simulink library "nmc"  (R2017b)
settings: Solver=ode45  StartTime=0.0  StopTime=10.0  RelTol=1e-3
undefined symbols (not defined in the file or in its folder): GroundFunction, theta
libraries: simulink x1
settings Model: Creator=efx  LastModifiedBy=FluitR
settings DataIOCC: LimitDataPoints=on  SaveFormat=Array
settings OptimizationCC: BlockReduction=off  BooleanDataType=off  LifeSpan=inf
settings DebuggingCC: SaveWithParameterizedLinksMsg=none  UnderspecifiedInitializationDetection=Classic  MergeDetectMultiDrivingBlocksExec=none  SignalResolutionControl=TryResolveAllWithWarning  AllowSymbolicDim=off  StrictBusMsg=Warning  SFUnexpectedBacktrackingDiag=warning  SFNoUnconditionalDefaultTransitionDiag=warning  SFExecutionAtInitializationDiag=none
settings HardwareCC: ProdBitPerPointer=32  ProdBitPerSizeT=32  ProdBitPerPtrDiffT=32  ProdLargestAtomicFloat=None  ProdIntDivRoundTo=Undefined  ProdEndianess=Unspecified  ProdWordSize=32  ProdHWDeviceType=32-bit Generic  TargetUnknown=on
settings ModelReferenceCC: PropagateSignalLabelsOutOfModel=off
settings CodeAppCC: StateflowObjectComments=on
settings GRTTargetCC: TargetLangStandard=C89/C90 (ANSI)  GeneratePreprocessorConditionals=Disable all
settings ConfigComp: CovMetricSettings=dw  CovHtmlReporting=on  CovSaveCumulativeToWorkspaceVar=on  CovSaveSingleToWorkspaceVar=on  CovExternalEMLEnable=off  CovSFcnEnable=off

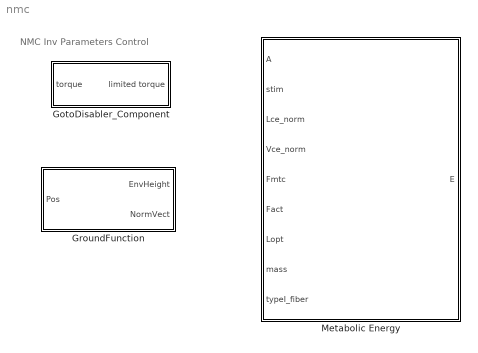
== system nmc ==
  note: NMC Inv Parameters Control
  GotoDisabler_Component : Subsystem  mask{GotoTag=DisableNMC_Component}
      mask prompts: GotoTag "Simulink:blkprm_prompts:FromGotoTag"
      mask TypeOptions GotoTag: From/GotoTag
      mask DialogControl GotoTag Prompt: Goto tag:
  GroundFunction : Subsystem
  Metabolic Energy : MATLAB Function  TreatAsAtomicUnit=on

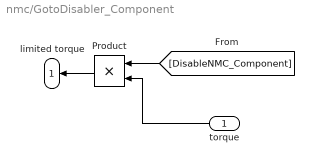
== system nmc/GotoDisabler_Component ==
  torque : Inport
  Product : Product
  limited torque : Outport
  wires:
  [DisableNMC_Component] -> Product/1
  Product/1 -> limited torque/1
  torque/1 -> Product/2

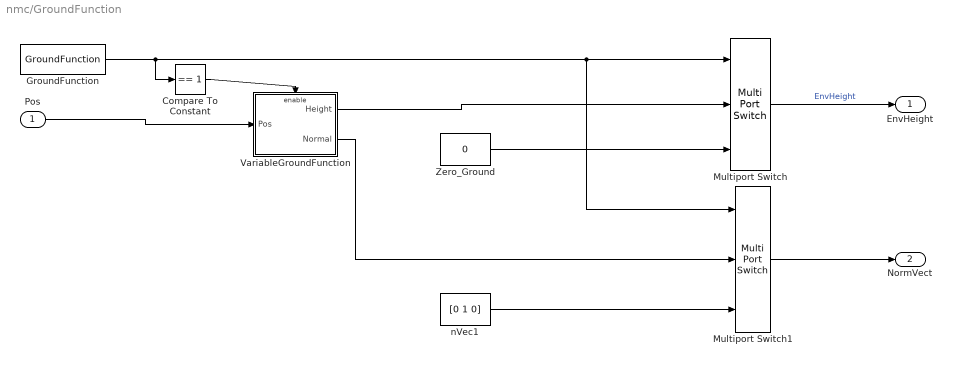
== system nmc/GroundFunction ==
  Pos : Inport
  Compare To Constant : simulink/Logic and Bit Operations/Compare To Constant  relop===  const=1  OutDataTypeStr=boolean  ZeroCross=off
  GroundFunction : Constant  Value=GroundFunction
  Multiport Switch : MultiPortSwitch  Inputs=2
  Multiport Switch1 : MultiPortSwitch  Inputs=2
  VariableGroundFunction : Subsystem
  Zero_Ground : Constant  Value=0
  nVec1 : Constant  Value=[0 1 0]
  EnvHeight : Outport
  NormVect : Outport  Port=2
  wires:
  GroundFunction/1 -> Compare To Constant/1, Multiport Switch1/1, Multiport Switch/1
  nVec1/1 -> Multiport Switch1/3
  Zero_Ground/1 -> Multiport Switch/3
  Multiport Switch1/1 -> NormVect/1
  Multiport Switch/1 -> EnvHeight/1  "EnvHeight"
  VariableGroundFunction/1(Height) -> Multiport Switch/2
  VariableGroundFunction/2(Normal) -> Multiport Switch1/2
  Pos/1 -> VariableGroundFunction/1(Pos)
  Compare To Constant/1 -> VariableGroundFunction/Enable

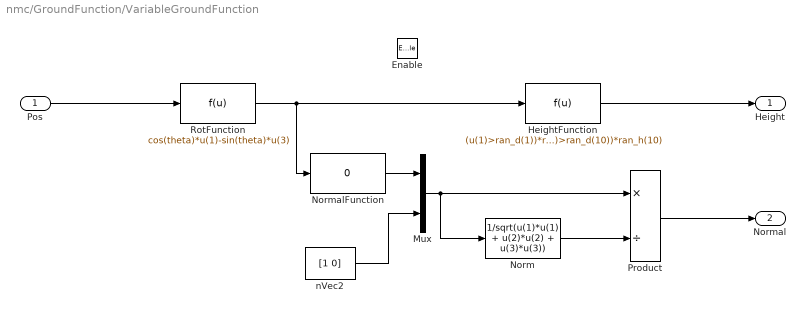
== system nmc/GroundFunction/VariableGroundFunction ==
  Pos : Inport
  Enable : EnablePort  ZeroCross=off
  HeightFunction : Fcn  Expr=(u(1)>ran_d(1))*ran_h(1)+(u(1)>ran_d(2))*ran_h(2)+(u(1)>ran_d(3))*ran_h(3)+(u(1)>ran_d(4))*ran_h(4)+(u(1)>ran_d(5))*ran_h(5)+(u(1)>ran_d(6))*ran_h(6)+(u(1)>ran_d(7))*ran_h(7)+(u(1)>ran_d(8))*ran_h(8)+(u(1)>ran_d(9))*ran_h(9)+(u(1)>ran_d(10))*ran_h(10)
  Mux : Mux  Inputs=2
  Norm : Fcn  Expr=1/sqrt(u(1)*u(1) + u(2)*u(2) + u(3)*u(3))
  NormalFunction : Fcn  Expr=0
  Product : Product  Inputs=*/
  RotFunction : Fcn  Expr=cos(theta)*u(1)-sin(theta)*u(3)
  nVec2 : Constant  Value=[1 0]
  Height : Outport
  Normal : Outport  Port=2
  wires:
  RotFunction/1 -> HeightFunction/1, NormalFunction/1
  Pos/1 -> RotFunction/1
  Product/1 -> Normal/1
  Mux/1 -> Product/1, Norm/1
  nVec2/1 -> Mux/2
  NormalFunction/1 -> Mux/1
  HeightFunction/1 -> Height/1
  Norm/1 -> Product/2

== matlab function nmc/Metabolic Energy ==
  data: A input; E output; stim input; Lce_norm input; Vce_norm input; Fmtc input; Fact input; Lopt input; mass input; typeI_fiber input
function E = MetaEnergy(A,stim,Lce_norm,Vce_norm,Fmtc,Fact,Lopt,mass,typeI_fiber)
%% Getting g
l = Lce_norm;
Vce = Vce_norm*Lopt;

g=zeros(length(l),1);

for i_l = 1:length(l)
    if l(i_l) >= 0 && l(i_l)  <= 0.5
        g(i_l) = 0.5;
    elseif l(i_l) > 0.5 && l(i_l) <= 1.0
        g(i_l) =  l(i_l) ;
    elseif(l(i_l) > 1.0 && l(i_l) <= 1.5)
        g(i_l) = -2*l(i_l) +3;
    else
        g(i_l) = 0;
    end
end

fM = 74 * typeI_fiber * sin(pi/2 * A) + 111*(1 - typeI_fiber).*(1-cos(pi/2* stim));
fA = 40 * typeI_fiber * sin(pi/2 * stim) + 133*(1 - typeI_fiber).*(1-cos(pi/2* stim));

energyM = mass.*g.*fM;
energyA = mass.*fA;
if -Vce > 0 %Velocity contractile element
    energyS =  0.25.*Fmtc.*(-Vce);
    energyW =  Fact.*(-Vce);
    
else
    energyS = 0;
    energyW = 0;
end

E = energyA + energyM + energyS + energyW;
end
